simulink model "tarea_1_cain"  (R2025a)
settings: Solver=VariableStepAuto  StartTime=0.0  StopTime=25  RelTol=1e-3
model workspace (MAT data in the model file):
  Beq = 4.3
  Bp = 0.0024
  Fc = 0
  Ip = 0.0079
  Lp = 0.3302
  Mc = 0.7031
  Mp = 0.23
  a = 0.0174533
  ader = 0
  g = 9.81
  xc = 0
  xcder = 0
settings Model: Creator=ISMAEL  LastModifiedBy=ismae

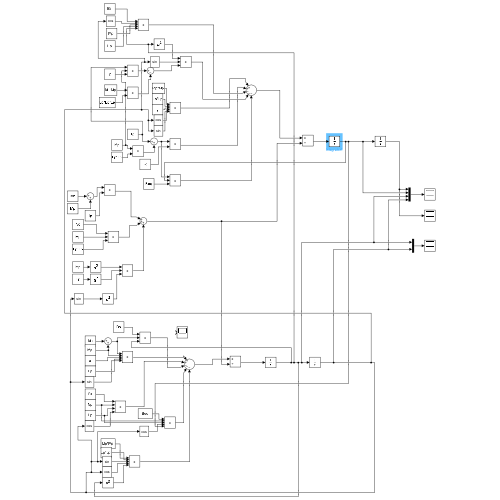
[thumbnail: Simulink's stored preview of the top-level diagram]
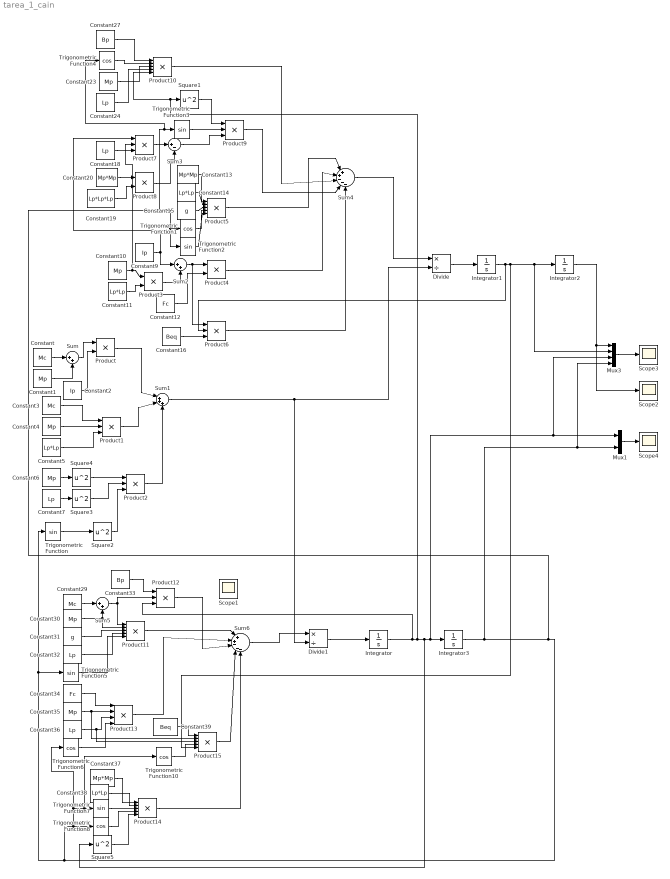
== system tarea_1_cain ==
  Constant : Constant  Value=Mc
  Constant{1,4,6,10,23,30,35} (7 alike) : Constant  Value=Mp
  Constant{5,11,14,38} (4 alike) : Constant  Value=Lp*Lp
  Constant12 : Constant  Value=Fc
  Constant13 : Constant  Value=Mp*Mp
  Constant15 : Constant  Value=g
  Constant16 : Constant  Value=Beq
  Constant{7,18,24,32,36} (5 alike) : Constant  Value=Lp
  Constant19 : Constant  Value=Lp*Lp*Lp
  Constant2 : Constant  Value=Ip
  Constant20 : Constant  Value=Mp*Mp
  Constant27 : Constant  Value=Bp
  Constant29 : Constant  Value=Mc
  Constant3 : Constant  Value=Mc
  Constant31 : Constant  Value=g
  Constant33 : Constant  Value=Bp
  Constant34 : Constant  Value=Fc
  Constant37 : Constant  Value=Mp*Mp
  Constant39 : Constant  Value=Beq
  Constant9 : Constant  Value=Ip
  Divide : Product  Inputs=*/
  Divide1 : Product  Inputs=*/
  Integrator : Integrator
  Integrator1 : Integrator
  Integrator2 : Integrator
  Integrator3 : Integrator  InitialCondition=0.017453
  Mux1 : Mux  Inputs=2
  Mux3 : Mux
  Product{,3..4,8} (4 alike) : Product
  Product{1..2,6..7,9,12} (6 alike) : Product  Inputs=3
  Product{5,10..11,14..15} (5 alike) : Product  Inputs=5
  Product13 : Product  Inputs=4
  Scope{1..4} (4 alike) : Scope
      Scope1 settings: ActiveDisplayYMinimum=-1.0904380973703272  ActiveDisplayYMaximum=0.8143238073915765
      Scope2 settings: ActiveDisplayYMinimum=-0.0090913383909884127  ActiveDisplayYMaximum=0.33682326379720068
      Scope3 settings: ActiveDisplayYMinimum=-12.779345390443106  ActiveDisplayYMaximum=42.923017152258929  DataLoggingVariableName=ScopeData3
      Scope4 settings: ActiveDisplayYMinimum=-617.03359314468889  ActiveDisplayYMaximum=725.0611390709455  DataLoggingVariableName=ScopeData2
  Square{1..5} (5 alike) : Math  Operator=square
  Sum : Sum  Inputs=|++
  Sum1 : Sum  Inputs=|+++
  Sum2 : Sum  Inputs=|++
  Sum3 : Sum  Inputs=|+-
  Sum4 : Sum  Inputs=|++---
  Sum5 : Sum  Inputs=|++
  Sum6 : Sum  Inputs=|++---
  Trigonometric Function{,2..3,5,7} (5 alike) : Trigonometry
  Trigonometric Function{1,4,6,8,10} (5 alike) : Trigonometry  Operator=cos
  wires:
  Constant/1 -> Sum/1
  Constant1/1 -> Sum/2
  Sum/1 -> Product/1
  Constant2/1 -> Product/2
  Constant3/1 -> Product1/1
  Constant4/1 -> Product1/2
  Constant5/1 -> Product1/3
  Trigonometric Function/1 -> Square2/1
  Constant6/1 -> Square4/1
  Constant7/1 -> Square3/1
  Square4/1 -> Product2/1
  Square3/1 -> Product2/2
  Square2/1 -> Product2/3
  Product/1 -> Sum1/1
  Product1/1 -> Sum1/2
  Product2/1 -> Sum1/3
  Constant10/1 -> Product3/1, Product7/2
  Constant11/1 -> Product3/2
  Product3/1 -> Sum2/2
  Sum2/1 -> Product4/1, Product6/1
  Constant12/1 -> Product4/2
  Constant13/1 -> Product5/1
  Constant14/1 -> Product5/2
  Constant15/1 -> Product5/3
  Trigonometric Function1/1 -> Product5/4
  Trigonometric Function2/1 -> Product5/5
  Constant16/1 -> Product6/3
  Constant9/1 -> Product7/1, Sum2/1
  Constant18/1 -> Product7/3
  Product7/1 -> Sum3/1
  Constant19/1 -> Product8/2
  Constant20/1 -> Product8/1
  Product8/1 -> Sum3/2
  Sum3/1 -> Product9/3
  Trigonometric Function3/1 -> Product9/2
  Square1/1 -> Product9/1
  Constant27/1 -> Product10/1
  Trigonometric Function4/1 -> Product10/2
  Constant23/1 -> Product10/3
  Constant24/1 -> Product10/4
  Product10/1 -> Sum4/3
  Product9/1 -> Sum4/4
  Product5/1 -> Sum4/1
  Product4/1 -> Sum4/2
  Product6/1 -> Sum4/5
  Sum4/1 -> Divide/1
  Sum1/1 -> Divide1/2, Divide/2
  Constant29/1 -> Sum5/1
  Constant30/1 -> Product11/2, Sum5/2
  Sum5/1 -> Product11/1, Product12/2
  Constant31/1 -> Product11/3
  Constant32/1 -> Product11/4
  Trigonometric Function5/1 -> Product11/5
  Constant33/1 -> Product12/1
  Integrator/1 -> Square5/1, Mux3/3, Mux1/1, Integrator3/1, Product10/5, Square1/1, Product12/3
  Constant34/1 -> Product13/1
  Constant35/1 -> Product15/2, Product13/2
  Constant36/1 -> Product15/3, Product13/3
  Trigonometric Function6/1 -> Product13/4
  Square5/1 -> Product14/5
  Trigonometric Function8/1 -> Product14/4
  Trigonometric Function7/1 -> Product14/3
  Constant38/1 -> Product14/2
  Constant37/1 -> Product14/1
  Trigonometric Function10/1 -> Product15/4
  Constant39/1 -> Product15/1
  Divide/1 -> Integrator1/1
  Product11/1 -> Sum6/1
  Product12/1 -> Sum6/3
  Product13/1 -> Sum6/2
  Product15/1 -> Sum6/4
  Product14/1 -> Sum6/5
  Sum6/1 -> Divide1/1
  Divide1/1 -> Integrator/1
  Mux1/1 -> Scope4/1
  Integrator3/1 -> Mux3/4, Mux1/2, Trigonometric Function2/1, Trigonometric Function1/1, Trigonometric Function4/1, Trigonometric Function3/1, Trigonometric Function/1, Trigonometric Function5/1, Trigonometric Function6/1, Trigonometric Function10/1, Trigonometric Function7/1, Trigonometric Function8/1
  Integrator1/1 -> Product6/2, Mux3/2, Integrator2/1, Product15/5
  Integrator2/1 -> Scope2/1, Mux3/1
  Mux3/1 -> Scope3/1
